simulink model "T1_R2015a"  (R2017b)
settings: Solver=VariableStepAuto  StartTime=0.0  StopTime=100  RelTol=1e-3
values from neighbouring files (symbols this model uses):
  B = 0.1    [Q1.m]
  didt0 = (-R/L)*i0-(Kw/L)*w0+(1/L)*V0    (= 0)    [Q1.m]
  dwdt0 = (-B/J)*w0-(1/J)*Tc0+(5.26/J)*exp(-i0)    [Q1.m]
  i0 = 0    [Q1.m]
  J = 1    [Q1.m]
  Kw = 1/3    (= 0.333333333333)    [Q1.m]
  L = 0.5    [Q1.m]
  R = 10    [Q1.m]
  Tc0 = 0    [Q1.m]
  V0 = 0    [Q1.m]
  w0 = 0    [Q1.m]
settings Model: Creator=VanderleiMunhozPerei  LastModifiedBy=VanderleiMunhozPerei

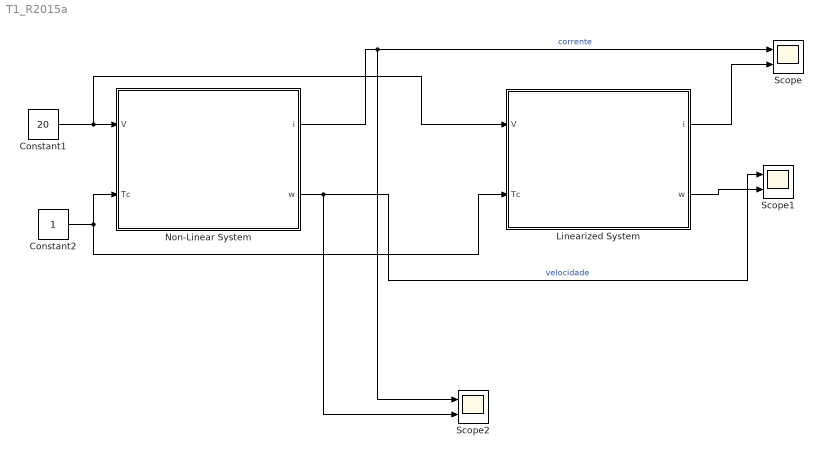
== system T1_R2015a ==
  Constant1 : Constant  Value=20
  Constant2 : Constant
  Linearized System : Subsystem
  Non-Linear System : Subsystem
  Scope : Scope  NumInputPorts=2
  Scope1 : Scope  NumInputPorts=2
  Scope2 : Scope  NumInputPorts=2
  wires:
  Constant1/1 -> Linearized System/1(V), Non-Linear System/1(V)
  Linearized System/1(i) -> Scope/2
  Constant2/1 -> Non-Linear System/2(Tc), Linearized System/2(Tc)
  Non-Linear System/2(w) -> Scope2/2, Scope1/1  "velocidade"
  Linearized System/2(w) -> Scope1/2
  Non-Linear System/1(i) -> Scope2/1, Scope/1  "corrente"

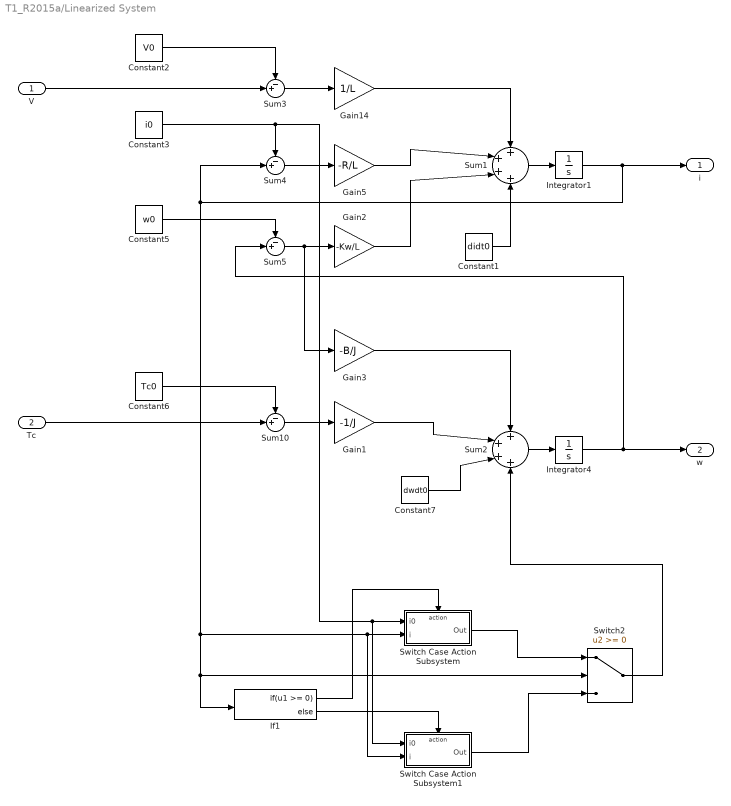
== system T1_R2015a/Linearized System ==
  V : Inport
  Tc : Inport  Port=2
  Constant1 : Constant  Value=didt0
  Constant2 : Constant  Value=V0
  Constant3 : Constant  Value=i0
  Constant5 : Constant  Value=w0
  Constant6 : Constant  Value=Tc0
  Constant7 : Constant  Value=dwdt0
  Gain1 : Gain  Gain=-1/J
  Gain14 : Gain  Gain=1/L
  Gain2 : Gain  Gain=-Kw/L
  Gain3 : Gain  Gain=-B/J
  Gain5 : Gain  Gain=-R/L
  If1 : If  IfExpression=u1 >= 0
  Integrator1 : Integrator
  Integrator4 : Integrator
  Sum1 : Sum  Inputs=+|+|+|+
  Sum{3..5,10} (4 alike) : Sum  Inputs=-+|
  Sum2 : Sum  Inputs=+|+|+|+
  Switch Case Action Subsystem : Subsystem  TreatAsAtomicUnit=on
  Switch Case Action Subsystem1 : Subsystem  TreatAsAtomicUnit=on
  Switch2 : Switch
  i : Outport
  w : Outport  Port=2
  wires:
  Switch Case Action Subsystem1/1(Out) -> Switch2/3
  Sum5/1 -> Gain3/1, Gain2/1
  Sum4/1 -> Gain5/1
  Sum1/1 -> Integrator1/1
  Gain5/1 -> Sum1/2
  Gain2/1 -> Sum1/3
  Tc/1 -> Sum10/2
  Sum3/1 -> Gain14/1
  Constant2/1 -> Sum3/1
  Gain3/1 -> Sum2/1
  Integrator4/1 -> w/1, Sum5/2
  Constant5/1 -> Sum5/1
  Sum10/1 -> Gain1/1
  Gain14/1 -> Sum1/1
  Gain1/1 -> Sum2/2
  If1/2 -> Switch Case Action Subsystem1/Action
  Constant6/1 -> Sum10/1
  Sum2/1 -> Integrator4/1
  V/1 -> Sum3/2
  Switch2/1 -> Sum2/4
  Constant7/1 -> Sum2/3
  Constant1/1 -> Sum1/4
  If1/1 -> Switch Case Action Subsystem/Action
  Constant3/1 -> Switch Case Action Subsystem1/1(i0), Switch Case Action Subsystem/1(i0), Sum4/1
  Integrator1/1 -> i/1, Switch Case Action Subsystem1/2(i), Switch Case Action Subsystem/2(i), If1/1, Switch2/2, Sum4/2
  Switch Case Action Subsystem/1(Out) -> Switch2/1

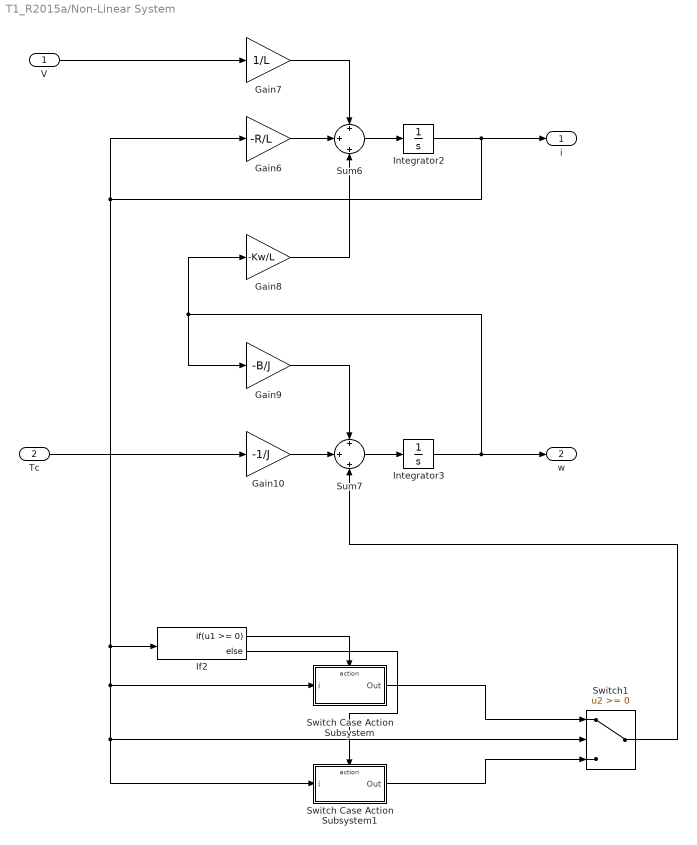
== system T1_R2015a/Non-Linear System ==
  V : Inport
  Tc : Inport  Port=2
  Gain10 : Gain  Gain=-1/J
  Gain6 : Gain  Gain=-R/L
  Gain7 : Gain  Gain=1/L
  Gain8 : Gain  Gain=-Kw/L
  Gain9 : Gain  Gain=-B/J
  If2 : If  IfExpression=u1 >= 0
  Integrator2 : Integrator
  Integrator3 : Integrator
  Sum6 : Sum  Inputs=+|+|+
  Sum7 : Sum  Inputs=+|+|+
  Switch Case Action Subsystem : Subsystem  TreatAsAtomicUnit=on
  Switch Case Action Subsystem1 : Subsystem  TreatAsAtomicUnit=on
  Switch1 : Switch
  i : Outport
  w : Outport  Port=2
  wires:
  Sum7/1 -> Integrator3/1
  Sum6/1 -> Integrator2/1
  Integrator3/1 -> w/1, Gain9/1, Gain8/1
  Gain7/1 -> Sum6/1
  Integrator2/1 -> i/1, Gain6/1, Switch1/2, Switch Case Action Subsystem1/1(i), Switch Case Action Subsystem/1(i), If2/1
  Gain9/1 -> Sum7/1
  Gain10/1 -> Sum7/2
  Switch1/1 -> Sum7/3
  Gain8/1 -> Sum6/3
  V/1 -> Gain7/1
  If2/1 -> Switch Case Action Subsystem/Action
  Gain6/1 -> Sum6/2
  Tc/1 -> Gain10/1
  If2/2 -> Switch Case Action Subsystem1/Action
  Switch Case Action Subsystem/1(Out) -> Switch1/1
  Switch Case Action Subsystem1/1(Out) -> Switch1/3

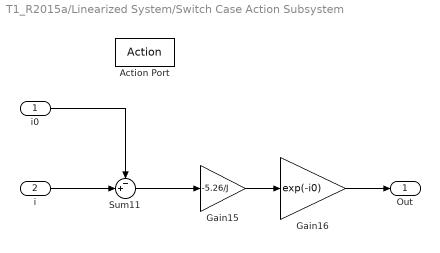
== system T1_R2015a/Linearized System/Switch Case Action Subsystem ==
  i0 : Inport
  i : Inport  Port=2
  Action Port : ActionPort  ActionType=then
  Gain15 : Gain  Gain=-5.26/J
  Gain16 : Gain  Gain=exp(-i0)
  Sum11 : Sum  Inputs=-+|
  Out : Outport
  wires:
  i0/1 -> Sum11/1
  Gain15/1 -> Gain16/1
  Sum11/1 -> Gain15/1
  i/1 -> Sum11/2
  Gain16/1 -> Out/1

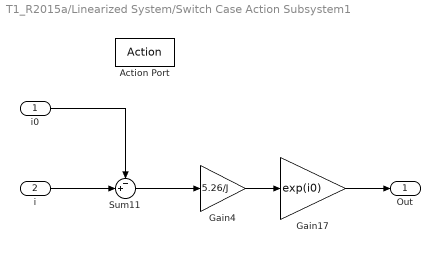
== system T1_R2015a/Linearized System/Switch Case Action Subsystem1 ==
  i0 : Inport
  i : Inport  Port=2
  Action Port : ActionPort  ActionType=else
  Gain17 : Gain  Gain=exp(i0)
  Gain4 : Gain  Gain=5.26/J
  Sum11 : Sum  Inputs=-+|
  Out : Outport
  wires:
  i0/1 -> Sum11/1
  i/1 -> Sum11/2
  Gain17/1 -> Out/1
  Gain4/1 -> Gain17/1
  Sum11/1 -> Gain4/1

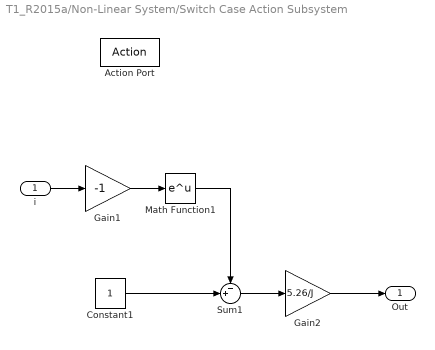
== system T1_R2015a/Non-Linear System/Switch Case Action Subsystem ==
  i : Inport
  Action Port : ActionPort  ActionType=then
  Constant1 : Constant
  Gain1 : Gain  Gain=-1
  Gain2 : Gain  Gain=5.26/J
  Math Function1 : Math  SaturateOnIntegerOverflow=on
  Sum1 : Sum  Inputs=-+|
  Out : Outport
  wires:
  Math Function1/1 -> Sum1/1
  i/1 -> Gain1/1
  Constant1/1 -> Sum1/2
  Sum1/1 -> Gain2/1
  Gain2/1 -> Out/1
  Gain1/1 -> Math Function1/1

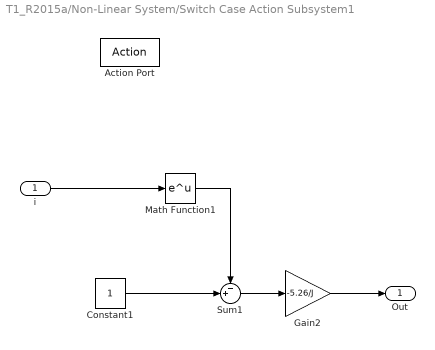
== system T1_R2015a/Non-Linear System/Switch Case Action Subsystem1 ==
  i : Inport
  Action Port : ActionPort  ActionType=else
  Constant1 : Constant
  Gain2 : Gain  Gain=-5.26/J
  Math Function1 : Math  SaturateOnIntegerOverflow=on
  Sum1 : Sum  Inputs=-+|
  Out : Outport
  wires:
  Math Function1/1 -> Sum1/1
  Constant1/1 -> Sum1/2
  Sum1/1 -> Gain2/1
  Gain2/1 -> Out/1
  i/1 -> Math Function1/1
